simulink model "hw_ukf_est_4para_myrobot"  (R2020b)
settings: Solver=ode1  StartTime=0.0  StopTime=60  FixedStep=0.01  RelTol=1e-3  EnableMultiTasking=on
libraries: arduinolib x4, simulink x2
settings Model: SILPILModeSetting=veronly  ExtModeTrigDuration=2  Creator=Sarot PC  LastModifiedBy=ONLY-GOD
settings OptimizationCC: EnhancedBackFolding=on  PassReuseOutputArgsAs=Individual arguments  ZeroExternalMemoryAtStartup=off  ZeroInternalMemoryAtStartup=off  MaxStackSize=64  OptimizeBlockOrder=speed  DifferentSizesBufferReuse=on  OptimizationCustomize=off  EfficientTunableParamExpr=on
settings DebuggingCC: ParameterTunabilityLossMsg=error
settings HardwareCC: ProdBitPerPointer=32  ProdBitPerSizeT=32  ProdBitPerPtrDiffT=32  ProdLargestAtomicInteger=Long  ProdLargestAtomicFloat=Double  ProdWordSize=32  ProdHWDeviceType=ARM Compatible->ARM Cortex
settings SFSimCC: MATLABDynamicMemAlloc=off
settings RTWCC: Description=Embedded Coder  SystemTargetFile=ert.tlc  HardwareBoard=Arduino Due  TemplateMakefile=ert_default_tmf  Toolchain=Arduino ARM  BuildConfiguration=Faster Runs
settings CodeAppCC: ForceParamTrailComments=on  IgnoreCustomStorageClasses=off  OperatorAnnotations=on  SimulinkDataObjDesc=on  SFDataObjDesc=on  InsertBlockDesc=on
settings ERTTargetCC: SupportContinuousTime=on  SupportVariableSizeSignals=on  ExtModeTransport=3  ExtModeStaticAllocSize=24576  ExtModeMexFile=ext_xcp  ExtModeIntrfLevel=Level2 - Open

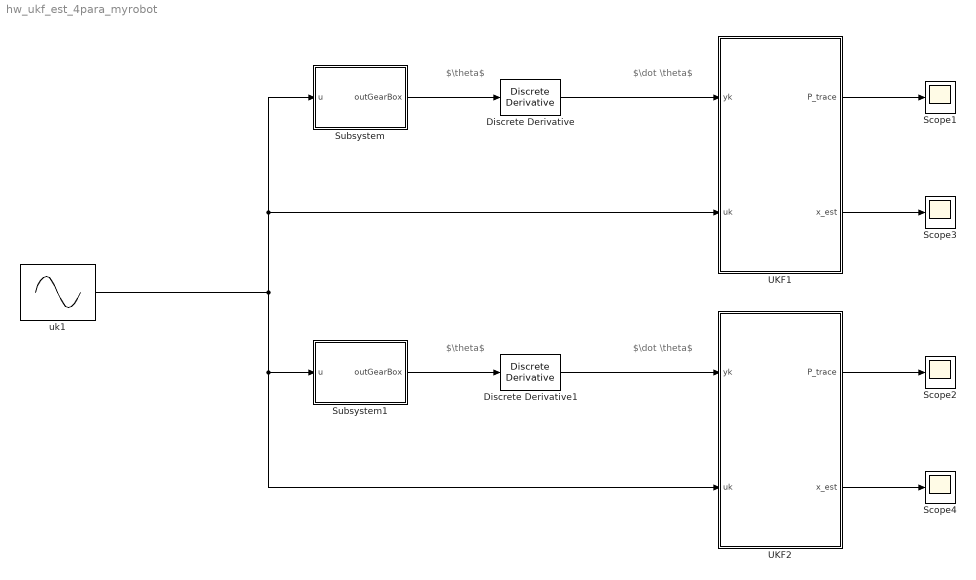
== system hw_ukf_est_4para_myrobot ==
  note: $\theta$
  note: $\dot \theta$
  note: $\theta$
  note: $\dot \theta$
  Discrete Derivative : simulink/Discrete/Discrete Derivative  gainval=1.0  ICPrevScaledInput=0.0  OutMin=[]  OutMax=[]  OutDataType=fixdt(1, 16)  OutScaling=2^-10  DoSatur=off
  Discrete Derivative1 : simulink/Discrete/Discrete Derivative  gainval=1.0  ICPrevScaledInput=0.0  OutMin=[]  OutMax=[]  OutDataType=fixdt(1, 16)  OutScaling=2^-10  DoSatur=off
  Scope{1..4} (4 alike) : Scope
  Subsystem : Subsystem
  Subsystem1 : Subsystem
  UKF1 : MATLAB Function  TreatAsAtomicUnit=on
  UKF2 : MATLAB Function  TreatAsAtomicUnit=on
  uk1 : Sin  Amplitude=20  Frequency=2*pi*0.1  SampleTime=0
  wires:
  Subsystem/1(outGearBox) -> Discrete Derivative/1
  uk1/1 -> UKF2/2(uk), Subsystem1/1(u), Subsystem/1(u), UKF1/2(uk)
  UKF1/1(P_trace) -> Scope1/1
  Discrete Derivative/1 -> UKF1/1(yk)
  UKF1/2(x_est) -> Scope3/1
  UKF2/2(x_est) -> Scope4/1
  Discrete Derivative1/1 -> UKF2/1(yk)
  UKF2/1(P_trace) -> Scope2/1
  Subsystem1/1(outGearBox) -> Discrete Derivative1/1

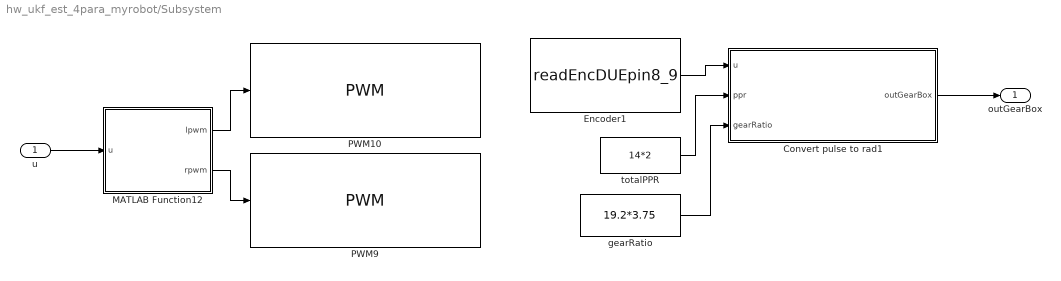
== system hw_ukf_est_4para_myrobot/Subsystem ==
  u : Inport
  Convert pulse to rad1 : MATLAB Function  TreatAsAtomicUnit=on
  Encoder1 : S-Function  InitFcn=try, set_param(gcb,'FunctionName','readEncDUEpin8_9'), end  FunctionName=readEncDUEpin8_9  SFunctionModules=readEncDUEpin8_9_wrapper  SFunctionDeploymentMode=off  EnableBusSupport=off  mask(S-Function Builder){}
      mask help: Simulink:masks:SFunctionBuilder_MD
      mask init:
      | val = [[.9  0.75 0.75 1 1 .9 .9 1]',[1 1 0.75 0.75 .9 .9 1 .9]'];try , sys = get_param(gcb,'SfunBuilderFcnName');if isempty(sys), sys = get_param(gcb,'FunctionName'); end,catch, sys = get_param(gcb,'FunctionName'); end
      settings: CopyFcn=set_param(gcbh,'LinkStatus','none')  PreSaveFcn=try, set_param(gcb,'FunctionName','readEncDUEpin8_9'), end  OpenFcn=sfunctionwizard(gcbh)
      mask Display: plot(val(:,1),val(:,2)),disp(sys),port_label('output',1,'count')
  MATLAB Function12 : MATLAB Function  TreatAsAtomicUnit=on
  PWM10 : arduinolib/PWM  pinNumber=7  frequencyType=Default  desiredFrequency=490.2  achievableFrequency=490.2
  PWM9 : arduinolib/PWM  pinNumber=6  frequencyType=Default  desiredFrequency=490.2  achievableFrequency=490.2
  gearRatio : Constant  Value=19.2*3.75
  totalPPR : Constant  Value=14*2
  outGearBox : Outport
  wires:
  Encoder1/1 -> Convert pulse to rad1/1(u)
  MATLAB Function12/1(lpwm) -> PWM10/1
  totalPPR/1 -> Convert pulse to rad1/2(ppr)
  MATLAB Function12/2(rpwm) -> PWM9/1
  gearRatio/1 -> Convert pulse to rad1/3(gearRatio)
  u/1 -> MATLAB Function12/1(u)
  Convert pulse to rad1/1(outGearBox) -> outGearBox/1

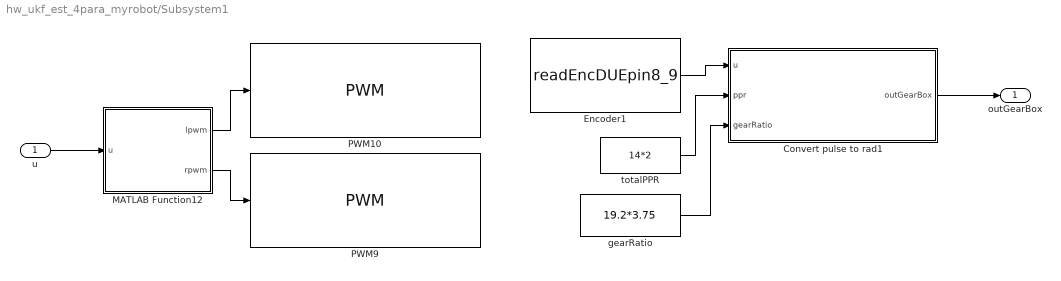
== system hw_ukf_est_4para_myrobot/Subsystem1 ==
  u : Inport
  Convert pulse to rad1 : MATLAB Function  TreatAsAtomicUnit=on
  Encoder1 : S-Function  InitFcn=try, set_param(gcb,'FunctionName','readEncDUEpin8_9'), end  FunctionName=readEncDUEpin8_9  SFunctionModules=readEncDUEpin8_9_wrapper  SFunctionDeploymentMode=off  EnableBusSupport=off  mask(S-Function Builder){}
      mask help: Simulink:masks:SFunctionBuilder_MD
      mask init: same as hw_ukf_est_4para_myrobot/Subsystem/Encoder1
      settings: CopyFcn=set_param(gcbh,'LinkStatus','none')  PreSaveFcn=try, set_param(gcb,'FunctionName','readEncDUEpin8_9'), end  OpenFcn=sfunctionwizard(gcbh)
      mask Display: plot(val(:,1),val(:,2)),disp(sys),port_label('output',1,'count')
  MATLAB Function12 : MATLAB Function  TreatAsAtomicUnit=on
  PWM10 : arduinolib/PWM  pinNumber=7  frequencyType=Default  desiredFrequency=490.2  achievableFrequency=490.2
  PWM9 : arduinolib/PWM  pinNumber=6  frequencyType=Default  desiredFrequency=490.2  achievableFrequency=490.2
  gearRatio : Constant  Value=19.2*3.75
  totalPPR : Constant  Value=14*2
  outGearBox : Outport
  wires:
  Convert pulse to rad1/1(outGearBox) -> outGearBox/1
  u/1 -> MATLAB Function12/1(u)
  gearRatio/1 -> Convert pulse to rad1/3(gearRatio)
  MATLAB Function12/2(rpwm) -> PWM9/1
  totalPPR/1 -> Convert pulse to rad1/2(ppr)
  MATLAB Function12/1(lpwm) -> PWM10/1
  Encoder1/1 -> Convert pulse to rad1/1(u)

== matlab function hw_ukf_est_4para_myrobot/Subsystem1/Convert pulse to rad1 ==
  settings: updateMethod=DISCRETE
  data: u input; ppr input; gearRatio input; outGearBox output
function outGearBox = fcn(u,ppr,gearRatio)

persistent counter_num over_flag
if(isempty(counter_num)), counter_num = 0;end
if(isempty(over_flag)), over_flag = 0;end
pulse2radian = 2*pi/ppr; % 1 pulse = ?? radian

if(double(u) - counter_num > 40000), over_flag = over_flag-1;
elseif(double(u) - counter_num < -40000), over_flag = over_flag+1;
end

inGearBox = (double(u)+over_flag*(2^32 -1))*pulse2radian; 
outGearBox = inGearBox/gearRatio;
counter_num = double(u) ;

== matlab function hw_ukf_est_4para_myrobot/Subsystem1/MATLAB Function12 ==
  data: u input; lpwm output; rpwm output
function [lpwm,rpwm] = fcn(u)

Vmax = 22.9;
pwm = u*254/Vmax;
if pwm > 0
    lpwm = pwm;
    rpwm = 0;
elseif pwm < 0
    lpwm = 0;
    rpwm = abs(pwm);
else
    lpwm = 0;
    rpwm = 0;
end

== matlab function hw_ukf_est_4para_myrobot/UKF2 ==
  data: P_trace output; x_est output; yk input size=[1,1]; uk input
function [P_trace,x_est] = fcn(yk,uk)
Ts = 0.01;
Qc = 1e-6*diag([0.1;0.1;15;10]);
R = 0.000002;
persistent n m xk1 Pk1 wm W lambda nsigma
n = 4; % number of state
m = 1; % number of output

if isempty(xk1)
    xk1= randn(n,1);
    Pk1 = 1e-1*eye(n);
    nsigma = 2*n+1;
    k=2;
    alpha=0.5;
    beta=1;
    lambda=alpha^2*(n+k)-n;
    Wm0=lambda/(n+lambda);
    Wc0=lambda/((n+lambda)+(1-alpha^2+beta));
    Wmi=1/2/(n+lambda);
    Wci=Wmi;
    wm=Wmi*ones(nsigma,1); wm(1)=Wm0;
    W=(eye(nsigma)-wm*ones(1,nsigma))*diag([Wc0 Wci*ones(1,2*n)])*(eye(nsigma)-wm*ones(1,nsigma))';
end


%Measurement Update
%Generate Sigma Points
x = xk1;
P = Pk1;
A   = chol(P,'lower');
X   = x*ones(1,nsigma) + sqrt(n+lambda)*[zeros(n,1) A -A];
Y   = zeros(m,nsigma);
for i=1:nsigma
    Y(:,i)= hd(uk,X(:,i));
end
y   = Y*wm;
Pxy = X*W*Y';
Pyy = Y*W*Y'+R;
K   = Pxy/Pyy;
x   = x + K*(yk-y);
P   = P - K*Pyy*K';

%Time Update
%Generate Sigma Points
A = chol(P,'lower');
X = x*ones(1,nsigma) + sqrt(n+lambda)*[zeros(n,1) A -A];
Xk1 = zeros(n,nsigma);
for i=1:nsigma
    Xk1(:,i)= fd(uk,X(:,i),Ts);
end
xk1     = Xk1*wm;
Pk1     = Xk1*W*Xk1'+Qc*Ts;
x_est   = xk1(1:4,1);
P_trace = trace(Pk1);
end

function y = hd(~,x)
C = [1,0,0,0];
y = C*x;
end

% Customizable function fc for various equation
function xk1 = fd(u,x,Ts)
x_dot = zeros(4,1);
x_dot(1,1) = -x(1,1)*x(2,1) + x(3,1)*u-x(4,1)*sign(x(1,1));
x_dot(2,1) = 0;
x_dot(3,1) = 0;
x_dot(4,1) = 0;
% end

% Discretization
xk1 = x + x_dot*Ts;
end

== matlab function hw_ukf_est_4para_myrobot/Subsystem/MATLAB Function12 ==
  data: u input; lpwm output; rpwm output
function [lpwm,rpwm] = fcn(u)

Vmax = 22.9;
pwm = u*254/Vmax;
if pwm > 0
    lpwm = pwm;
    rpwm = 0;
elseif pwm < 0
    lpwm = 0;
    rpwm = abs(pwm);
else
    lpwm = 0;
    rpwm = 0;
end

== matlab function hw_ukf_est_4para_myrobot/UKF1 ==
  data: P_trace output; x_est output; yk input size=[1,1]; uk input
function [P_trace,x_est] = fcn(yk,uk)
Ts = 0.01;
Qc = 1e-6*diag([0.1;0.1;15;10]);
R = 0.000002;
persistent n m xk1 Pk1 wm W lambda nsigma
n = 4; % number of state
m = 1; % number of output

if isempty(xk1)
    xk1= randn(n,1);
    Pk1 = 1e-1*eye(n);
    nsigma = 2*n+1;
    k=2;
    alpha=0.5;
    beta=1;
    lambda=alpha^2*(n+k)-n;
    Wm0=lambda/(n+lambda);
    Wc0=lambda/((n+lambda)+(1-alpha^2+beta));
    Wmi=1/2/(n+lambda);
    Wci=Wmi;
    wm=Wmi*ones(nsigma,1); wm(1)=Wm0;
    W=(eye(nsigma)-wm*ones(1,nsigma))*diag([Wc0 Wci*ones(1,2*n)])*(eye(nsigma)-wm*ones(1,nsigma))';
end


%Measurement Update
%Generate Sigma Points
x = xk1;
P = Pk1;
A   = chol(P,'lower');
X   = x*ones(1,nsigma) + sqrt(n+lambda)*[zeros(n,1) A -A];
Y   = zeros(m,nsigma);
for i=1:nsigma
    Y(:,i)= hd(uk,X(:,i));
end
y   = Y*wm;
Pxy = X*W*Y';
Pyy = Y*W*Y'+R;
K   = Pxy/Pyy;
x   = x + K*(yk-y);
P   = P - K*Pyy*K';

%Time Update
%Generate Sigma Points
A = chol(P,'lower');
X = x*ones(1,nsigma) + sqrt(n+lambda)*[zeros(n,1) A -A];
Xk1 = zeros(n,nsigma);
for i=1:nsigma
    Xk1(:,i)= fd(uk,X(:,i),Ts);
end
xk1     = Xk1*wm;
Pk1     = Xk1*W*Xk1'+Qc*Ts;
x_est   = xk1(1:4,1);
P_trace = trace(Pk1);
end

function y = hd(~,x)
C = [1,0,0,0];
y = C*x;
end

% Customizable function fc for various equation
function xk1 = fd(u,x,Ts)
x_dot = zeros(4,1);
x_dot(1,1) = -x(1,1)*x(2,1) + x(3,1)*u-x(4,1)*sign(x(1,1));
x_dot(2,1) = 0;
x_dot(3,1) = 0;
x_dot(4,1) = 0;
% end

% Discretization
xk1 = x + x_dot*Ts;
end

== matlab function hw_ukf_est_4para_myrobot/Subsystem/Convert pulse to rad1 ==
  settings: updateMethod=DISCRETE
  data: u input; ppr input; gearRatio input; outGearBox output
function outGearBox = fcn(u,ppr,gearRatio)

persistent counter_num over_flag
if(isempty(counter_num)), counter_num = 0;end
if(isempty(over_flag)), over_flag = 0;end
pulse2radian = 2*pi/ppr; % 1 pulse = ?? radian

if(double(u) - counter_num > 40000), over_flag = over_flag-1;
elseif(double(u) - counter_num < -40000), over_flag = over_flag+1;
end

inGearBox = (double(u)+over_flag*(2^32 -1))*pulse2radian; 
outGearBox = inGearBox/gearRatio;
counter_num = double(u) ;
